simulink model "Overtaking_Integrated"  (R2020b)
settings: Solver=ode23tb  StartTime=0.0  StopTime=25  FixedStep=.01  RelTol=5e-3  EnableMultiTasking=on
InitFcn:
  | %SimulationParameters;
StartFcn:
  | %tic
StopFcn:
  | %toc
  | save(['SimOutputs\' char(datetime('now','Format','y_M_d_HH_mm_ss')) '_' 'sim_out.mat'], 'logsout');
model workspace (MAT data in the model file):
  DLCXref = [-3.2158 4.0142 4.2842 14.7842 29.7842 30.2842 41.7842 46.7842 56.7842]
  DLCYref = [-3.1012 -3.1012 -7.6012 -7.1012 -6.8512 -1.6012 -1.8512 -3.1012 -3.1012]
  Downshift_Speeds = [9.5625 12.9375 16.3125 19.6875 23.0625 26.4375 29.8125 33.1875 36.5625 39.9375 43.3125 46.6875 ... (28 elements, 4x7)]
  EngRevLim = 7000
  Pedal_Positions = [0.1 0.4 0.5 0.9]
  Upshift_Speeds = [12.9375 16.3125 19.6875 33 26.4375 29.8125 33.1875 52.5 39.9375 43.3125 46.6875 77.25 ... (28 elements, 4x7)]
  VEH : object (value not decoded)
values from neighbouring files (symbols this model uses):
  abortTrigger = 0.0    [AOTDataDictionary.sldd]
  Dmax = 3.0    [AOTDataDictionary.sldd]
  dt = 0.05    [AOTDataDictionary.sldd]
  egoVehLength = 4.948    [AOTDataDictionary.sldd]
  egoVehWidth = 2.009    [AOTDataDictionary.sldd]
  gamma = 0.5    [AOTDataDictionary.sldd]
  inflationFactor = 1.1    [AOTDataDictionary.sldd]
  inflexPoint = 0.0    [AOTDataDictionary.sldd]
  L = 3.705    [AOTDataDictionary.sldd]
  npcVehLength = 4.848    [AOTDataDictionary.sldd]
  npcVehWidth = 1.842    [AOTDataDictionary.sldd]
  plotSampleTime = 0.1    [AOTDataDictionary.sldd]
  SenseResolution = 0.1    [AOTDataDictionary.sldd]
  XSenseRange = 20.0    [AOTDataDictionary.sldd]
  YSenseRange = 20.0    [AOTDataDictionary.sldd]
symbols that are objects in the model workspace (value not decoded): VEH
undefined symbols (not defined in the file or in its folder): driving
libraries: simulink x10, drivingscenarioandsensors x5, autolibutils x4, sim3dautolib x3, sim3dlib x2, autolibshared x1, vehdynlibdriver x1, vehdynlibscenariocommon x1, pid_lib x1, vehdynlibsens x1
(part 2 of 3)

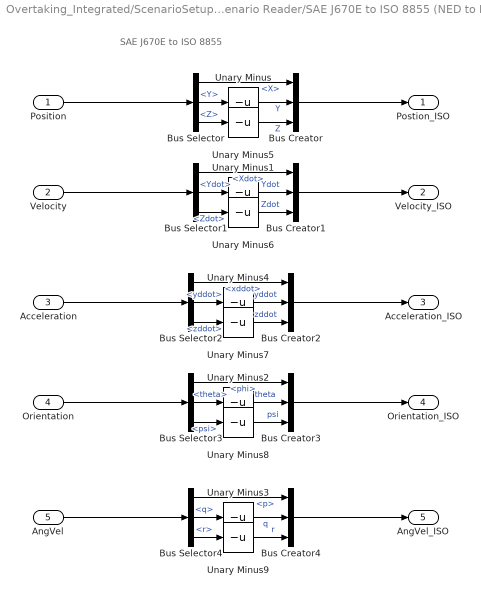
== system Overtaking_Integrated/ScenarioSetup/Scenario Reader/SAE J670E to ISO 8855 (NED to NWU)1 ==
  note: SAE J670E to ISO 8855
  Position : Inport  Unit=m
  Velocity : Inport  Port=2  Unit=m/s
  Acceleration : Inport  Port=3  Unit=m/s^2
  Orientation : Inport  Port=4  Unit=rad
  AngVel : Inport  Port=5  Unit=rad/s
  Bus Creator{,1..4} (5 alike) : BusCreator  Inputs=3
  Bus Selector : BusSelector  OutputSignals=X,Y,Z
  Bus Selector1 : BusSelector  OutputSignals=Xdot,Ydot,Zdot
  Bus Selector2 : BusSelector  OutputSignals=xddot,yddot,zddot
  Bus Selector3 : BusSelector  OutputSignals=phi,theta,psi
  Bus Selector4 : BusSelector  OutputSignals=p,q,r
  Unary Minus{,1..9} (10 alike) : UnaryMinus
  Postion_ISO : Outport  Unit=m  VectorParamsAs1DForOutWhenUnconnected=off
  Velocity_ISO : Outport  Port=2  Unit=m/s  VectorParamsAs1DForOutWhenUnconnected=off  LockScale=on
  Acceleration_ISO : Outport  Port=3  Unit=m/s^2  VectorParamsAs1DForOutWhenUnconnected=off
  Orientation_ISO : Outport  Port=4  Unit=rad  VectorParamsAs1DForOutWhenUnconnected=off
  AngVel_ISO : Outport  Port=5  Unit=rad/s  VectorParamsAs1DForOutWhenUnconnected=off
  wires:
  Bus Creator2/1 -> Acceleration_ISO/1
  Position/1 -> Bus Selector/1
  Bus Selector/2 -> Unary Minus/1  "<Y>"
  Bus Selector/1 -> Bus Creator/1  "<X>"
  Unary Minus/1 -> Bus Creator/2  "Y"
  Bus Selector/3 -> Unary Minus5/1  "<Z>"
  Unary Minus5/1 -> Bus Creator/3  "Z"
  Bus Creator/1 -> Postion_ISO/1
  Unary Minus6/1 -> Bus Creator1/3  "Zdot"
  Unary Minus1/1 -> Bus Creator1/2  "Ydot"
  Bus Selector1/2 -> Unary Minus1/1  "<Ydot>"
  Bus Selector1/1 -> Bus Creator1/1  "<Xdot>"
  Bus Selector1/3 -> Unary Minus6/1  "<Zdot>"
  Velocity/1 -> Bus Selector1/1
  Bus Creator1/1 -> Velocity_ISO/1
  Unary Minus7/1 -> Bus Creator2/3  "zddot"
  Unary Minus4/1 -> Bus Creator2/2  "yddot"
  Bus Selector2/2 -> Unary Minus4/1  "<yddot>"
  Bus Selector2/1 -> Bus Creator2/1  "<xddot>"
  Bus Selector2/3 -> Unary Minus7/1  "<zddot>"
  Acceleration/1 -> Bus Selector2/1
  Bus Selector3/3 -> Unary Minus8/1  "<psi>"
  Bus Selector3/2 -> Unary Minus2/1  "<theta>"
  Unary Minus2/1 -> Bus Creator3/2  "theta"
  Bus Selector3/1 -> Bus Creator3/1  "<phi>"
  Unary Minus8/1 -> Bus Creator3/3  "psi"
  Orientation/1 -> Bus Selector3/1
  Bus Creator3/1 -> Orientation_ISO/1
  Bus Selector4/1 -> Bus Creator4/1  "<p>"
  Bus Creator4/1 -> AngVel_ISO/1
  Bus Selector4/2 -> Unary Minus3/1  "<q>"
  Unary Minus9/1 -> Bus Creator4/3  "r"
  Unary Minus3/1 -> Bus Creator4/2  "q"
  Bus Selector4/3 -> Unary Minus9/1  "<r>"
  AngVel/1 -> Bus Selector4/1

== system Overtaking_Integrated/Subsystem3/Driver Commands/Driver Commands ==
  VehRef : Inport
  VehFdbk : Inport  Port=2
  SteerCmd : Inport  Port=3
  Accel : Inport  Port=4
  Brake : Inport  Port=5
  Gear : Inport  Port=6
  Longitudinal Driver : Subsystem  VariantControl=0
  Open Loop Constant Radius : Subsystem  VariantControl=2
  Predictive Driver : Subsystem  VariantControl=1
  " Driver" : Outport  VectorParamsAs1DForOutWhenUnconnected=off

== system Overtaking_Integrated/Vehicle Plant/Controllers/Active Differential Control ==
  note: 1) Add Subsystem or Model blocks as valid variant choices.
      | 2) You cannot connect blocks at this level. At simulation, connectivity is automatically
      | determined, based on the active variant and port name matching.
  Accel : Inport
  BrkCmd : Inport  Port=2
  Steer : Inport  Port=3
  GearFdbk : Inport  Port=4
  Omega : Inport  Port=5  Unit=rad/s
  axayaz : Inport  Port=6
  pqr : Inport  Port=7
  No Control : Subsystem  VariantControl=0
  Rear Diff Controller : Subsystem  TreatAsAtomicUnit=on  SystemSampleTime=.01  VariantControl=1
  DiffPrsCmd : Outport  VectorParamsAs1DForOutWhenUnconnected=off
  TrqCmd : Outport  Port=2  VectorParamsAs1DForOutWhenUnconnected=off

== system Overtaking_Integrated/Vehicle Plant/Controllers/Brake Controller ==
  BrkCmd : Inport
  Omega : Inport  Port=2
  kappa : Inport  Port=3
  Abs : Abs  ZeroCross=off
  Brake Pressure Control : Subsystem  Variant=on  VariantControlMode=label  LabelModeActiveChoice=0
  Constant1 : Constant  Value=-20
  Gain3 : Gain
  Integrator2 : Integrator  LimitOutput=on  UpperSaturationLimit=1  LowerSaturationLimit=0
  Saturation : Saturate  UpperLimit=1  LowerLimit=0  ZeroCross=off
  Switch1 : Switch  Criteria=u2 > Threshold  Threshold=.1
  Vector Concatenate2 : Concatenate  NumInputs=4
  BrkPrsCmd : Outport  VectorParamsAs1DForOutWhenUnconnected=off
  wires:
  Constant1/1 -> Switch1/3
  Gain3/1 -> Switch1/1
  Saturation/1 -> Brake Pressure Control/3(<Kappa>)  "Kappa"
  Brake Pressure Control/1(BrkPrsCmd) -> BrkPrsCmd/1
  kappa/1 -> Abs/1
  Integrator2/1 -> Vector Concatenate2/4, Vector Concatenate2/3, Vector Concatenate2/2, Vector Concatenate2/1
  Omega/1 -> Brake Pressure Control/2(Omega)
  Abs/1 -> Saturation/1
  Vector Concatenate2/1 -> Brake Pressure Control/1(Pref)  "Reference P"
  BrkCmd/1 -> Switch1/2, Gain3/1
  Switch1/1 -> Integrator2/1

== system Overtaking_Integrated/Vehicle Plant/Controllers/ECU ==
  DiffTrqCmd : Inport
  <Accel> : Inport  Port=2
  EngSpd : Inport  Port=3
  First Order Hold : FirstOrderHold  ErrorTolerance=100
  Torque Cmd : Subsystem  TreatAsAtomicUnit=on  SystemSampleTime=.01
  EngTrqCmd : Outport  VectorParamsAs1DForOutWhenUnconnected=off
  wires:
  First Order Hold/1 -> EngTrqCmd/1
  DiffTrqCmd/1 -> Torque Cmd/1(DiffTrqCmd)
  <Accel>/1 -> Torque Cmd/2(<Accel>)
  EngSpd/1 -> Torque Cmd/3(EngSpd)
  Torque Cmd/1(EngTrqCmd) -> First Order Hold/1

== system Overtaking_Integrated/Vehicle Plant/Controllers/Transmission Controller ==
  Accel : Inport
  BrkCmd : Inport  Port=2
  GearReq : Inport  Port=3
  EngSpd : Inport  Port=4
  Omega : Inport  Port=5  Unit=rad/s
  UpReq : Inport  Port=6
  DownReq : Inport  Port=7  Unit=rad/s
  Driver - No Clutch : Subsystem  VariantControl=1
  PRNDL Controller : Subsystem  VariantControl=3
  Paddles : Subsystem  VariantControl=2
  Transmission Controller : Subsystem  VariantControl=0
  " Gear" : Outport  VectorParamsAs1DForOutWhenUnconnected=off

== system Overtaking_Integrated/Vehicle Plant/Environment/Ground Feedback ==
  Friction : Inport
  3D Engine : Subsystem  VariantControl=1
  Constant : Subsystem  VariantControl=0
  Ground : Outport  VectorParamsAs1DForOutWhenUnconnected=off

== system Overtaking_Integrated/Vehicle Plant/Passenger Vehicle/Body, Suspension, Wheels ==
  note: 1) Add Subsystem or Model blocks as valid variant choices.
      | 2) You cannot connect blocks at this level. At simulation, connectivity is automatically
      | determined, based on the active variant and port name matching.
  WindXYZ : Inport
  Ground : Inport  Port=2  PortDimensions=4
  Friction : Inport  Port=3  PortDimensions=4
  WhlAng : Inport  Port=4
  AxlTrq : Inport  Port=5
  BrkPrs : Inport  Port=6
  PassVeh14DOF : ModelReference  DisableCoverage=on  ModelNameDialog=PassVeh14DOF  VariantControl=3  ModelReferenceVersion=2.28
  PassVeh7DOF : ModelReference  ModelNameDialog=PassVeh7DOF  SimulationMode=Normal  VariantControl=1  ModelReferenceVersion=2.94
  Veh : Outport  VectorParamsAs1DForOutWhenUnconnected=off
  Wheels : Outport  Port=2  VectorParamsAs1DForOutWhenUnconnected=off

== system Overtaking_Integrated/Vehicle Plant/Passenger Vehicle/Chassis Input ==
  Env : Inport
  Driveline : Inport  Port=2
  Bus Selector1 : BusSelector  OutputSignals=Gnd.z.G_FL_z,Gnd.z.G_FR_z,Gnd.z.G_RL_z,Gnd.z.G_RR_z
  Bus Selector2 : BusSelector  OutputSignals=Wind
  Bus Selector3 : BusSelector  OutputSignals=Gnd.mu.mu_FL,Gnd.mu.mu_FR,Gnd.mu.mu_RL,Gnd.mu.mu_RR
  Bus Selector4 : BusSelector  OutputSignals=WhlAng,AxlTrq,BrkPrs
  Vector Concatenate : Concatenate  NumInputs=4
  Vector Concatenate1 : Concatenate  NumInputs=4
  Wind : Outport  VectorParamsAs1DForOutWhenUnconnected=off
  Gnd : Outport  Port=2  VectorParamsAs1DForOutWhenUnconnected=off
  mu : Outport  Port=3  VectorParamsAs1DForOutWhenUnconnected=off
  WhlAng : Outport  Port=4  VectorParamsAs1DForOutWhenUnconnected=off
  AxlTrq : Outport  Port=5  VectorParamsAs1DForOutWhenUnconnected=off
  BrkPrs : Outport  Port=6  VectorParamsAs1DForOutWhenUnconnected=off
  wires:
  Env/1 -> Bus Selector3/1, Bus Selector1/1, Bus Selector2/1
  Bus Selector2/1 -> Wind/1  "<Wind>"
  Bus Selector3/1 -> Vector Concatenate/1  "<mu_FL>"
  Bus Selector3/2 -> Vector Concatenate/2  "<mu_FR>"
  Bus Selector3/3 -> Vector Concatenate/3  "<mu_RL>"
  Bus Selector3/4 -> Vector Concatenate/4  "<mu_RR>"
  Vector Concatenate/1 -> mu/1
  Bus Selector1/1 -> Vector Concatenate1/1  "<G_FL_z>"
  Bus Selector1/2 -> Vector Concatenate1/2  "<G_FR_z>"
  Bus Selector1/3 -> Vector Concatenate1/3  "<G_RL_z>"
  Bus Selector1/4 -> Vector Concatenate1/4  "<G_RR_z>"
  Vector Concatenate1/1 -> Gnd/1
  Driveline/1 -> Bus Selector4/1
  Bus Selector4/2 -> AxlTrq/1  "<AxlTrq>"
  Bus Selector4/1 -> WhlAng/1  "<WhlAng>"
  Bus Selector4/3 -> BrkPrs/1  "<BrkPrs>"

== system Overtaking_Integrated/Vehicle Plant/Passenger Vehicle/Chassis Output ==
  Veh : Inport
  Wheels : Inport  Port=2
  Out Bus Element4 : Outport  PortName=VehFdbk
  Out Bus Element1 : Outport  Port=2  PortName=WheelsFdbk
  wires:
  Veh/1 -> Out Bus Element4/1
  Wheels/1 -> Out Bus Element1/1

== system Overtaking_Integrated/Vehicle Plant/Passenger Vehicle/Driveline Input ==
  Cntrl : Inport
  Driver : Inport  Port=2
  EngTrqCmd : Inport  Port=3
  Wheels : Inport  Port=4
  Bus Selector1 : BusSelector  OutputSignals=SteerCmd
  Bus Selector2 : BusSelector  OutputSignals=TireFrame.Omega
  Bus Selector3 : BusSelector  OutputSignals=Transmission.GearCmd,Brake.BrkPrsCmd,Diff.DiffPrsCmd
  Bus Selector4 : BusSelector  OutputSignals=EngTrq
  Data Type Conversion : DataTypeConversion
  Steer : Outport  VectorParamsAs1DForOutWhenUnconnected=off
  EngTrq : Outport  Port=2  VectorParamsAs1DForOutWhenUnconnected=off
  GearCmd : Outport  Port=3  VectorParamsAs1DForOutWhenUnconnected=off
  BrkPrsCmd : Outport  Port=4  VectorParamsAs1DForOutWhenUnconnected=off
  Omega : Outport  Port=5  VectorParamsAs1DForOutWhenUnconnected=off
  DiffPrsCmd : Outport  Port=6  VectorParamsAs1DForOutWhenUnconnected=off
  wires:
  Cntrl/1 -> Bus Selector3/1
  Bus Selector3/1 -> Data Type Conversion/1  "<GearCmd>"
  Driver/1 -> Bus Selector1/1
  Wheels/1 -> Bus Selector2/1
  Bus Selector2/1 -> Omega/1  "<Omega>"
  Bus Selector3/2 -> BrkPrsCmd/1  "<BrkPrsCmd>"
  EngTrqCmd/1 -> Bus Selector4/1
  Bus Selector1/1 -> Steer/1  "<SteerCmd>"
  Bus Selector4/1 -> EngTrq/1  "<EngTrq>"
  Bus Selector3/3 -> DiffPrsCmd/1  "<DiffPrsCmd>"
  Data Type Conversion/1 -> GearCmd/1

== system Overtaking_Integrated/Vehicle Plant/Passenger Vehicle/Driveline Output ==
  WhlAng : Inport
  AxlTrq : Inport  Port=2
  BrkPrs : Inport  Port=3
  EngSpd : Inport  Port=4
  PropShftSpd : Inport  Port=5
  StrWhlTrq : Inport  Port=6
  Gear : Inport  Port=7
  Bus Creator1 : BusCreator  Inputs=6
  Bus Creator2 : BusCreator  Inputs=1
  Driveline : Outport  VectorParamsAs1DForOutWhenUnconnected=off
  Steering : Outport  Port=2  VectorParamsAs1DForOutWhenUnconnected=off
  wires:
  Bus Creator1/1 -> Driveline/1  "Driveline"
  PropShftSpd/1 -> Bus Creator1/5  "PropShftSpd"
  AxlTrq/1 -> Bus Creator1/2  "AxlTrq"
  WhlAng/1 -> Bus Creator1/1  "WhlAng"
  EngSpd/1 -> Bus Creator1/4  "EngSpd"
  BrkPrs/1 -> Bus Creator1/3  "BrkPrs"
  StrWhlTrq/1 -> Bus Creator2/1  "StrWhlTrq"
  Bus Creator2/1 -> Steering/1  "Steering"
  Gear/1 -> Bus Creator1/6  "Gear"

== system Overtaking_Integrated/Vehicle Plant/Passenger Vehicle/Engine ==
  note: 1) Add Subsystem or Model blocks as valid variant choices.
      | 2) You cannot connect blocks at this level. At simulation, connectivity is automatically
      | determined, based on the active variant and port name matching.
  TrqCmd : Inport
  EngSpd : Inport  Port=2  Unit=rad/s
  Ideal Mapped Engine : ModelReference  DisableCoverage=on  ModelNameDialog=SiMappedEngineV  VariantControl=0  ModelReferenceVersion=1.335
  EngTrq : Outport  VectorParamsAs1DForOutWhenUnconnected=off

== system Overtaking_Integrated/Vehicle Plant/Passenger Vehicle/Engine Input ==
  Cntrl : Inport
  Driveline : Inport  Port=2
  Bus Selector : BusSelector  OutputSignals=ECU.EngTrqCmd
  Bus Selector1 : BusSelector  OutputSignals=EngSpd
  EngTrqCmd : Outport  VectorParamsAs1DForOutWhenUnconnected=off
  EngSpd : Outport  Port=2  VectorParamsAs1DForOutWhenUnconnected=off
  wires:
  Driveline/1 -> Bus Selector1/1
  Cntrl/1 -> Bus Selector/1
  Bus Selector/1 -> EngTrqCmd/1  "<EngTrqCmd>"
  Bus Selector1/1 -> EngSpd/1  "<EngSpd>"

== system Overtaking_Integrated/Vehicle Plant/Passenger Vehicle/Engine Output ==
  "EngTrq " : Inport
  Bus Creator : BusCreator  Inputs=1
  Eng : Outport  VectorParamsAs1DForOutWhenUnconnected=off
  wires:
  "EngTrq "/1 -> Bus Creator/1  "EngTrq"
  Bus Creator/1 -> Eng/1

== system Overtaking_Integrated/Vehicle Plant/Passenger Vehicle/Pedal Cluster Input ==
  Driver : Inport
  Driveline : Inport  Port=2
  Steering : Inport  Port=3
  Bus Selector : BusSelector  OutputSignals=SteerCmd,AccelCmd,DecelCmd,GearCmd
  Bus Selector1 : BusSelector  OutputSignals=BrkPrs
  Bus Selector2 : BusSelector  OutputSignals=StrWhlTrq
  SteerCmd : Outport  VectorParamsAs1DForOutWhenUnconnected=off
  AccelCmd : Outport  Port=2  VectorParamsAs1DForOutWhenUnconnected=off
  DecelCmd : Outport  Port=3  VectorParamsAs1DForOutWhenUnconnected=off
  GearCmd : Outport  Port=4  VectorParamsAs1DForOutWhenUnconnected=off
  BrkPrs : Outport  Port=5  VectorParamsAs1DForOutWhenUnconnected=off
  StrWhlTrq : Outport  Port=6  VectorParamsAs1DForOutWhenUnconnected=off
  wires:
  Bus Selector/2 -> AccelCmd/1  "<AccelCmd>"
  Driver/1 -> Bus Selector/1
  Bus Selector/3 -> DecelCmd/1  "<DecelCmd>"
  Bus Selector/4 -> GearCmd/1  "<GearCmd>"
  Bus Selector/1 -> SteerCmd/1  "<SteerCmd>"
  Driveline/1 -> Bus Selector1/1
  Bus Selector1/1 -> BrkPrs/1  "<BrkPrs>"
  Steering/1 -> Bus Selector2/1
  Bus Selector2/1 -> StrWhlTrq/1  "<StrWhlTrq>"

== system Overtaking_Integrated/Vehicle Plant/Passenger Vehicle/Pedal Cluster Output ==
  SteerFdbk : Inport
  AccFdbk : Inport  Port=2
  DecelFdbk : Inport  Port=3
  GearFdbk : Inport  Port=4
  Bus Creator1 : BusCreator  Inputs=4
  Signal Specification : SignalSpecification  Unit=rad
  Signal Specification1 : SignalSpecification  Unit=1
  Signal Specification2 : SignalSpecification  Unit=1
  Signal Specification3 : SignalSpecification  Unit=1
  OperatorFdbk : Outport
  wires:
  Signal Specification1/1 -> Bus Creator1/2  "AccFdbk"
  Signal Specification3/1 -> Bus Creator1/4  "GearFdbk"
  AccFdbk/1 -> Signal Specification1/1
  DecelFdbk/1 -> Signal Specification2/1
  GearFdbk/1 -> Signal Specification3/1
  Signal Specification/1 -> Bus Creator1/1  "SteerFdbk"
  SteerFdbk/1 -> Signal Specification/1
  Bus Creator1/1 -> OperatorFdbk/1
  Signal Specification2/1 -> Bus Creator1/3  "DecelFdbk"

== system Overtaking_Integrated/Vehicle Plant/Passenger Vehicle/Pedal Cluster and Cabin ==
  note: Placeholder for introducing faults, detailed actuator behavior,
      | interactions of other systems with a human interface such
      | as changes in power steering and braking assistance.
  SteerCmd : Inport
  AccCmd : Inport  Port=2
  DecelCmd : Inport  Port=3
  GearCmd : Inport  Port=4
  BrkPrs : Inport  Port=5
  StrWhlTrq : Inport  Port=6
  Terminator : Terminator
  Terminator1 : Terminator
  SteerFdbk : Outport
  AccFdbk : Outport  Port=2
  DecelFdbk : Outport  Port=3
  GearFdbk : Outport  Port=4
  wires:
  SteerCmd/1 -> SteerFdbk/1
  AccCmd/1 -> AccFdbk/1
  DecelCmd/1 -> DecelFdbk/1
  GearCmd/1 -> GearFdbk/1
  BrkPrs/1 -> Terminator/1
  StrWhlTrq/1 -> Terminator1/1

== system Overtaking_Integrated/Vehicle Plant/Passenger Vehicle/Steering, Transmission, Driveline and Brakes ==
  note: 1) Add Subsystem or Model blocks as valid variant choices.
      | 2) You cannot connect blocks at this level. At simulation, connectivity is automatically
      | determined, based on the active variant and port name matching.
  SteerHWCmd : Inport
  EngTrq : Inport  Port=2
  GearCmd : Inport  Port=3  OutDataTypeStr=int8
  BrkPrsCmd : Inport  Port=4  PortDimensions=4
  Omega : Inport  Port=5
  DiffPrsCmd : Inport  Port=6
  Driveline Ideal Fixed Gear : ModelReference  DisableCoverage=on  ModelNameDialog=Driveline  VariantControl=0  ModelReferenceVersion=1.238
  WhlAng : Outport  VectorParamsAs1DForOutWhenUnconnected=off
  AxlTrq : Outport  Port=2  VectorParamsAs1DForOutWhenUnconnected=off
  BrkPrs : Outport  Port=3  PortDimensions=4  VectorParamsAs1DForOutWhenUnconnected=off
  EngSpd : Outport  Port=4  Unit=rad/s  VectorParamsAs1DForOutWhenUnconnected=off
  PropShftSpd : Outport  Port=5  VectorParamsAs1DForOutWhenUnconnected=off
  StrWhlTrq : Outport  Port=6  VectorParamsAs1DForOutWhenUnconnected=off
  Gear : Outport  Port=7  VectorParamsAs1DForOutWhenUnconnected=off

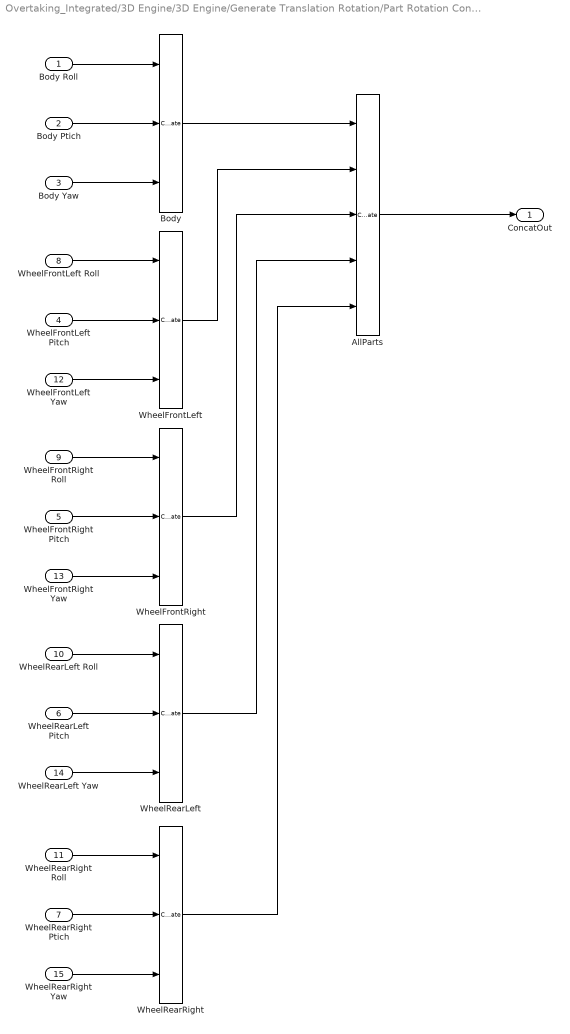
== system Overtaking_Integrated/3D Engine/3D Engine/Generate Translation Rotation/Part Rotation Concatenation ==
  Body Roll : Inport
  Body Ptich : Inport  Port=2
  Body Yaw : Inport  Port=3
  WheelFrontLeft Pitch : Inport  Port=4
  WheelFrontRight Pitch : Inport  Port=5
  WheelRearLeft Pitch : Inport  Port=6
  WheelRearRight Ptich : Inport  Port=7
  WheelFrontLeft Roll : Inport  Port=8
  WheelFrontRight Roll : Inport  Port=9
  WheelRearLeft Roll : Inport  Port=10
  WheelRearRight Roll : Inport  Port=11
  WheelFrontLeft Yaw : Inport  Port=12
  WheelFrontRight Yaw : Inport  Port=13
  WheelRearLeft Yaw : Inport  Port=14
  WheelRearRight Yaw : Inport  Port=15
  AllParts : Concatenate  NumInputs=5  Mode=Multidimensional array
  Body : Concatenate  NumInputs=3  Mode=Multidimensional array  ConcatenateDimension=2
  WheelFrontLeft : Concatenate  NumInputs=3  Mode=Multidimensional array  ConcatenateDimension=2
  WheelFrontRight : Concatenate  NumInputs=3  Mode=Multidimensional array  ConcatenateDimension=2
  WheelRearLeft : Concatenate  NumInputs=3  Mode=Multidimensional array  ConcatenateDimension=2
  WheelRearRight : Concatenate  NumInputs=3  Mode=Multidimensional array  ConcatenateDimension=2
  ConcatOut : Outport  VectorParamsAs1DForOutWhenUnconnected=off
  wires:
  Body Yaw/1 -> Body/3
  WheelFrontLeft Yaw/1 -> WheelFrontLeft/3
  WheelFrontLeft/1 -> AllParts/2
  Body/1 -> AllParts/1
  WheelRearLeft/1 -> AllParts/4
  WheelFrontRight/1 -> AllParts/3
  WheelRearRight Yaw/1 -> WheelRearRight/3
  WheelRearLeft Yaw/1 -> WheelRearLeft/3
  AllParts/1 -> ConcatOut/1
  WheelRearRight/1 -> AllParts/5
  WheelFrontRight Yaw/1 -> WheelFrontRight/3
  Body Roll/1 -> Body/1
  Body Ptich/1 -> Body/2
  WheelFrontLeft Pitch/1 -> WheelFrontLeft/2
  WheelFrontLeft Roll/1 -> WheelFrontLeft/1
  WheelFrontRight Roll/1 -> WheelFrontRight/1
  WheelFrontRight Pitch/1 -> WheelFrontRight/2
  WheelRearLeft Roll/1 -> WheelRearLeft/1
  WheelRearLeft Pitch/1 -> WheelRearLeft/2
  WheelRearRight Roll/1 -> WheelRearRight/1
  WheelRearRight Ptich/1 -> WheelRearRight/2

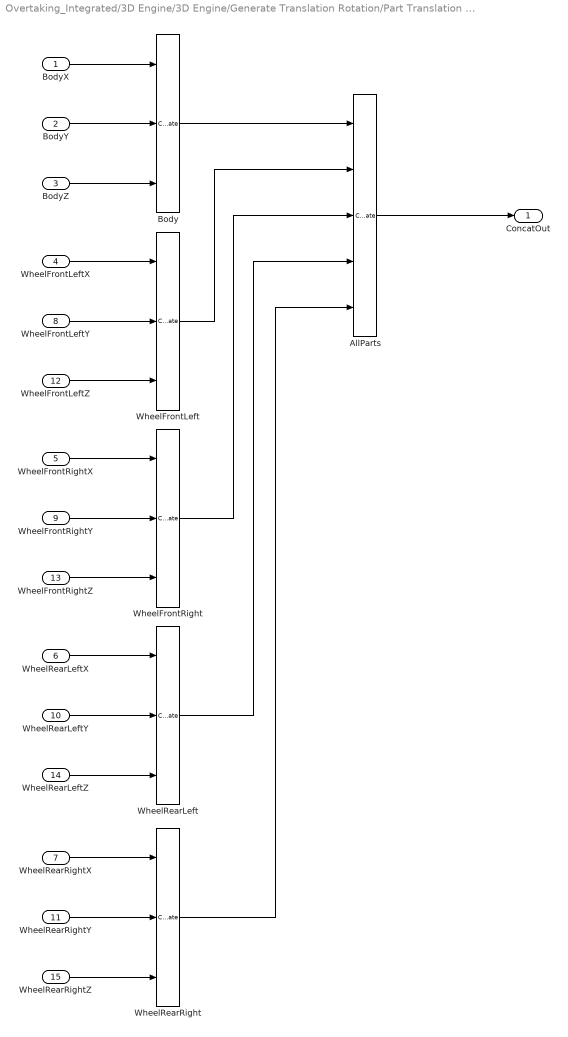
== system Overtaking_Integrated/3D Engine/3D Engine/Generate Translation Rotation/Part Translation Concatenation ==
  BodyX : Inport
  BodyY : Inport  Port=2
  BodyZ : Inport  Port=3
  WheelFrontLeftX : Inport  Port=4
  WheelFrontRightX : Inport  Port=5
  WheelRearLeftX : Inport  Port=6
  WheelRearRightX : Inport  Port=7
  WheelFrontLeftY : Inport  Port=8
  WheelFrontRightY : Inport  Port=9
  WheelRearLeftY : Inport  Port=10
  WheelRearRightY : Inport  Port=11
  WheelFrontLeftZ : Inport  Port=12
  WheelFrontRightZ : Inport  Port=13
  WheelRearLeftZ : Inport  Port=14
  WheelRearRightZ : Inport  Port=15
  AllParts : Concatenate  NumInputs=5  Mode=Multidimensional array
  Body : Concatenate  NumInputs=3  Mode=Multidimensional array  ConcatenateDimension=2
  WheelFrontLeft : Concatenate  NumInputs=3  Mode=Multidimensional array  ConcatenateDimension=2
  WheelFrontRight : Concatenate  NumInputs=3  Mode=Multidimensional array  ConcatenateDimension=2
  WheelRearLeft : Concatenate  NumInputs=3  Mode=Multidimensional array  ConcatenateDimension=2
  WheelRearRight : Concatenate  NumInputs=3  Mode=Multidimensional array  ConcatenateDimension=2
  ConcatOut : Outport  VectorParamsAs1DForOutWhenUnconnected=off
  wires:
  BodyX/1 -> Body/1
  BodyZ/1 -> Body/3
  WheelFrontLeftX/1 -> WheelFrontLeft/1
  WheelFrontLeftZ/1 -> WheelFrontLeft/3
  WheelFrontLeftY/1 -> WheelFrontLeft/2
  BodyY/1 -> Body/2
  WheelFrontLeft/1 -> AllParts/2
  WheelRearRightX/1 -> WheelRearRight/1
  Body/1 -> AllParts/1
  WheelRearLeft/1 -> AllParts/4
  WheelFrontRight/1 -> AllParts/3
  WheelRearRightZ/1 -> WheelRearRight/3
  WheelFrontRightY/1 -> WheelFrontRight/2
  WheelFrontRightX/1 -> WheelFrontRight/1
  WheelRearRightY/1 -> WheelRearRight/2
  WheelRearLeftZ/1 -> WheelRearLeft/3
  AllParts/1 -> ConcatOut/1
  WheelRearLeftY/1 -> WheelRearLeft/2
  WheelRearRight/1 -> AllParts/5
  WheelRearLeftX/1 -> WheelRearLeft/1
  WheelFrontRightZ/1 -> WheelFrontRight/3

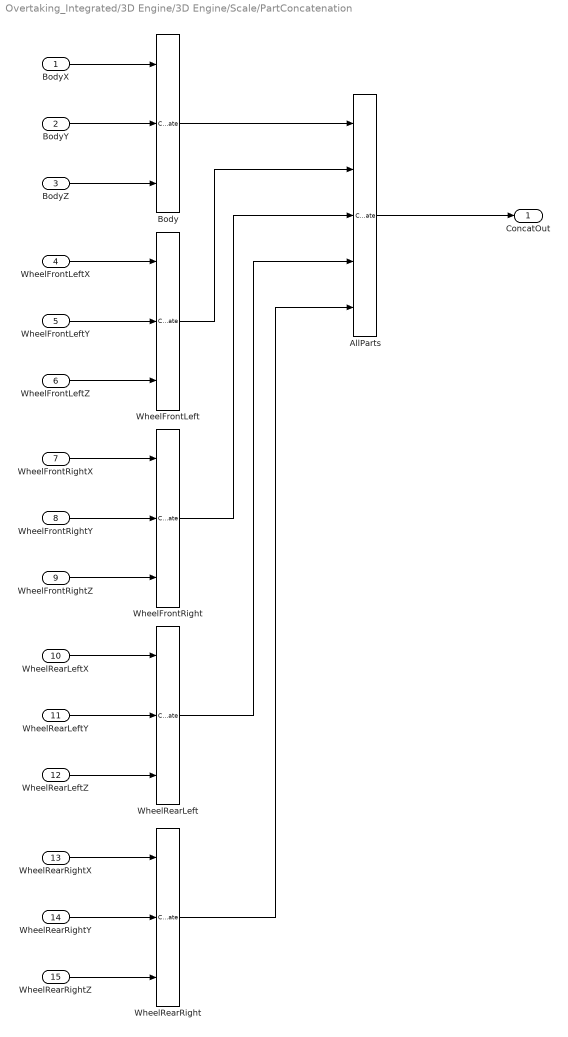
== system Overtaking_Integrated/3D Engine/3D Engine/Scale/PartConcatenation ==
  BodyX : Inport
  BodyY : Inport  Port=2
  BodyZ : Inport  Port=3
  WheelFrontLeftX : Inport  Port=4
  WheelFrontLeftY : Inport  Port=5
  WheelFrontLeftZ : Inport  Port=6
  WheelFrontRightX : Inport  Port=7
  WheelFrontRightY : Inport  Port=8
  WheelFrontRightZ : Inport  Port=9
  WheelRearLeftX : Inport  Port=10
  WheelRearLeftY : Inport  Port=11
  WheelRearLeftZ : Inport  Port=12
  WheelRearRightX : Inport  Port=13
  WheelRearRightY : Inport  Port=14
  WheelRearRightZ : Inport  Port=15
  AllParts : Concatenate  NumInputs=5  Mode=Multidimensional array
  Body : Concatenate  NumInputs=3  Mode=Multidimensional array  ConcatenateDimension=2
  WheelFrontLeft : Concatenate  NumInputs=3  Mode=Multidimensional array  ConcatenateDimension=2
  WheelFrontRight : Concatenate  NumInputs=3  Mode=Multidimensional array  ConcatenateDimension=2
  WheelRearLeft : Concatenate  NumInputs=3  Mode=Multidimensional array  ConcatenateDimension=2
  WheelRearRight : Concatenate  NumInputs=3  Mode=Multidimensional array  ConcatenateDimension=2
  ConcatOut : Outport  VectorParamsAs1DForOutWhenUnconnected=off
  wires:
  BodyX/1 -> Body/1
  BodyZ/1 -> Body/3
  WheelFrontLeftX/1 -> WheelFrontLeft/1
  WheelFrontLeftZ/1 -> WheelFrontLeft/3
  WheelFrontLeftY/1 -> WheelFrontLeft/2
  BodyY/1 -> Body/2
  WheelFrontLeft/1 -> AllParts/2
  WheelRearRightX/1 -> WheelRearRight/1
  Body/1 -> AllParts/1
  WheelRearLeft/1 -> AllParts/4
  WheelFrontRight/1 -> AllParts/3
  WheelRearRightZ/1 -> WheelRearRight/3
  WheelFrontRightY/1 -> WheelFrontRight/2
  WheelFrontRightX/1 -> WheelFrontRight/1
  WheelRearRightY/1 -> WheelRearRight/2
  WheelRearLeftZ/1 -> WheelRearLeft/3
  AllParts/1 -> ConcatOut/1
  WheelRearLeftY/1 -> WheelRearLeft/2
  WheelRearRight/1 -> AllParts/5
  WheelRearLeftX/1 -> WheelRearLeft/1
  WheelFrontRightZ/1 -> WheelFrontRight/3

== system Overtaking_Integrated/Subsystem3/Driver Commands/Driver Commands/Longitudinal Driver ==
  VehRef : Inport
  VehFdbk : Inport  Port=2
  Bus Creator2 : BusCreator  Inputs=5
  Bus Selector2 : BusSelector  OutputSignals=Body.BdyFrm.Cg.Vel.xdot,Body.InertFrm.Cg.Disp.X
  Bus Selector3 : BusSelector  OutputSignals=SteerOvrCmd,LngRef,LtrlRef
  Dead Zone1 : DeadZone  LowerValue=-.1  UpperValue=.1  SaturateOnIntegerOverflow=on
  Ground1 : Ground
  Ground2 : Ground
  Longitudinal Driver : autolibshared/Longitudinal Driver  extAccelOvr=off  extDecelOvr=off  extAccelHld=off  extDecelHld=off  extAccelZero=off  extDecelZero=off  cntrlType=Predictive  shftType=Reverse, Neutral, Drive  velUnits=m/s  gearOut=on  Kp=5  Ki=5  Kff=.1  Kg=0  VehVelVec=[0 100]  KffVec=[.1 .1]  KpVec=[10 10]  KiVec=[5 5]  KgVec=[0 0]  m=VEH.Mass  Kpt=3000  tau=.5  L=2  aR=200  bR=2.5  cR=.5  g=9.81  vnom=5  Kaw=1  tauerr=.1  tauPt=2  GearInit=0  tShift=.1  pdlVec=[0.1 0.4 0.5 0.9]  upShftTbl=[-1 12.9375 26.4375 39.9375 51.18749999999999 62.4375 72.84375 83.25;-1 16.3125 29.8125 43.3125 54.5624 65.8125 76.78125 87.75;-1 19.6875 33.1875 46.68749999999999 57.9375 69.1875 80.71875 92.25;-1 33 52.5 77.25 100.5 138.75 161.875 185]  dwnShftTbl=[1 9.5625 23.0625 36.5625 47.8125 59.0625 68.90625 78.75;1 12.9375 26.4375 39.9375 51.18749999999999 62.4375 72.84375 83.25;1 16.3125 29.8125 43.3125 54.562499 65.8125 76.78125 87.75;1 19.6875 33.1875 46.68749999999999 57.9375 69.1875 80.71875 92.25]  tClutch=.5  tRev=.5  tPark=120  aMode=2  UpGearVec="[0  1  2  3  4  5  6  7]"  DownGearVec="[1  2  3  4  5  6  7  8]"
      settings: SourceProductBaseCode=PW,MT,UV,VE,VP
  Mux : Mux  Inputs=3
  Signal Copy : SignalConversion  OverrideOpt=off
  Terminator1 : Terminator
  Driver : Outport  VectorParamsAs1DForOutWhenUnconnected=off
  wires:
  VehRef/1 -> Bus Selector3/1
  Signal Copy/1 -> Bus Creator2/1  "SteerCmd"
  Longitudinal Driver/2 -> Bus Creator2/2  "AccelCmd"
  Dead Zone1/1 -> Longitudinal Driver/2
  Bus Selector3/2 -> Longitudinal Driver/1  "<LngRef>"
  Ground1/1 -> Longitudinal Driver/3
  Bus Selector2/1 -> Dead Zone1/1  "<xdot>"
  Bus Creator2/1 -> Driver/1
  Longitudinal Driver/1 -> Terminator1/1
  Longitudinal Driver/3 -> Bus Creator2/3  "DecelCmd"
  VehFdbk/1 -> Bus Selector2/1
  Bus Selector3/1 -> Signal Copy/1  "<SteerOvrCmd>"
  Ground2/1 -> Mux/3
  Bus Selector2/2 -> Mux/1  "<X>"
  Mux/1 -> Bus Creator2/5  "Ref"
  Bus Selector3/3 -> Mux/2  "<LtrlRef>"
  Longitudinal Driver/4 -> Bus Creator2/4  "GearCmd"

== system Overtaking_Integrated/Subsystem3/Driver Commands/Driver Commands/Open Loop Constant Radius ==
  VehFdbk : Inport
  SteerCmd : Inport  Port=2
  Accel : Inport  Port=3  Unit=one
  Brake : Inport  Port=4  Unit=1
  Gear : Inport  Port=5  Unit=1
  Bus Creator1 : BusCreator  Inputs=4
  Signal Specification : SignalSpecification  Unit=rad
  Signal Specification1 : SignalSpecification  Unit=1
  Signal Specification2 : SignalSpecification  Unit=1
  Signal Specification3 : SignalSpecification  Unit=1
  Terminator : Terminator
  Unit Conversion{,1..3} (4 alike) : UnitConversion
  Driver : Outport  VectorParamsAs1DForOutWhenUnconnected=off
  wires:
  Unit Conversion3/1 -> Signal Specification3/1
  Unit Conversion2/1 -> Signal Specification2/1
  Unit Conversion/1 -> Signal Specification/1
  Bus Creator1/1 -> Driver/1
  Accel/1 -> Unit Conversion1/1
  VehFdbk/1 -> Terminator/1
  SteerCmd/1 -> Unit Conversion/1
  Unit Conversion1/1 -> Signal Specification1/1
  Brake/1 -> Unit Conversion2/1
  Gear/1 -> Unit Conversion3/1
  Signal Specification/1 -> Bus Creator1/1  "SteerCmd"
  Signal Specification1/1 -> Bus Creator1/2  "AccelCmd"
  Signal Specification2/1 -> Bus Creator1/3  "DecelCmd"
  Signal Specification3/1 -> Bus Creator1/4  "GearCmd"

== system Overtaking_Integrated/Subsystem3/Driver Commands/Driver Commands/Predictive Driver ==
  VehRef : Inport
  VehFdbk : Inport  Port=2
  Bus Creator1 : BusCreator  Inputs=5
  Bus Selector : BusSelector  OutputSignals=Body.BdyFrm.Cg.Vel.xdot,Body.InertFrm.Cg.Disp.Y,Body.BdyFrm.Cg.Vel.ydot,Body.InertFrm.Cg.Ang.psi,Body.BdyFrm.Cg.AngVel.r,Body.InertFrm.Cg.Disp.X
  Bus Selector1 : BusSelector  OutputSignals=LngRef,LtrlRef,EnblSteerCmd,SteerOvrCmd,AccelZero
  Dead Zone : DeadZone  LowerValue=-.5  UpperValue=.5  ZeroCross=off  SaturateOnIntegerOverflow=on
  Ground : Ground
  Ground1 : Ground
  Linear Predictive Driver : vehdynlibdriver/Predictive Driver  extAccelOvr=off  extDecelOvr=off  extAccelHld=off  extDecelHld=off  extAccelZero=on  extDecelZero=off  extSteerOvr=on  extSteerHld=off  extSteerZero=off  cntrlType=Predictive  cntrlTypeLat=Predictive  shftType=Reverse, Neutral, Drive  coordMode=SAE J670 (Z-down)  velUnits=m/s  angUnits=rad  gearOut=on  steerOut=on  Kp=3  Ki=1  Kff=1  Kg=0  VehVelVec=[0 100]  KffVec=[.1 .1]  KpVec=[10 10]  KiVec=[5 5]  KgVec=[0 0]  vnom=5  Kaw=1  tauerr=.075  tau=.15  L=6  Kpt=15000  aR=200  bR=2.5  cR=.5  g=9.81  vecPose=off  dynamMode=on  PositionGainF=2.5  PositionGainR=2.5  YawRateGain=.2  DelayGain=.2  a=VEH.FrontAxlePositionfromCG  b=VEH.RearAxlePositionfromCG  m=VEH.Mass  Cy_f=5000  Cy_r=7000  I=VEH.YawMomentInertia  Ksteer=18  theta=40*pi/180  GearInit=0  tShift=.1  pdlVec=[0.1 0.4 0.5 0.9]  upShftTbl=[-1 12.9375 26.4375 39.9375 51.18749999999999 62.4375 72.84375 83.25;-1 16.3125 29.8125 43.3125 54.5624 65.8125 76.78125 87.75;-1 19.6875 33.1875 46.68749999999999 57.9375 69.1875 80.71875 92.25;-1 33 52.5 77.25 100.5 138.75 161.875 185]  dwnShftTbl=[-1 12.9375 26.4375 39.9375 51.18749999999999 62.4375 72.84375 83.25;-1 16.3125 29.8125 43.3125 54.5624 65.8125 76.78125 87.75;-1 19.6875 33.1875 46.68749999999999 57.9375 69.1875 80.71875 92.25;-1 33 52.5 77.25 100.5 138.75 161.875 185]  tClutch=.5  tRev=.5  tPark=120  UpGearVec="[0  1  2  3  4  5  6  7]"  DownGearVec="[1  2  3  4  5  6  7  8]"  aMode=2
      settings: SourceProductBaseCode=VE
  Mux : Mux  Inputs=3
  Terminator : Terminator
  Driver : Outport  VectorParamsAs1DForOutWhenUnconnected=off
  wires:
  Mux/1 -> Bus Creator1/5  "Ref"
  Bus Selector/6 -> Mux/1  "<X>"
  Linear Predictive Driver/5 -> Bus Creator1/4  "GearCmd"
  Bus Selector/3 -> Linear Predictive Driver/9  "<ydot>"
  Linear Predictive Driver/1 -> Terminator/1
  Bus Selector/5 -> Linear Predictive Driver/11  "<r>"
  Bus Selector1/2 -> Mux/2, Linear Predictive Driver/2  "<LtrlRef>"
  Ground1/1 -> Mux/3
  Ground/1 -> Linear Predictive Driver/6
  Bus Selector/1 -> Dead Zone/1  "<xdot>"
  Bus Selector/4 -> Linear Predictive Driver/10  "<psi>"
  Linear Predictive Driver/4 -> Bus Creator1/3  "DecelCmd"
  Dead Zone/1 -> Linear Predictive Driver/7
  VehFdbk/1 -> Bus Selector/1
  VehRef/1 -> Bus Selector1/1  "xdotref"
  Linear Predictive Driver/2 -> Bus Creator1/1  "SteerCmd"
  Bus Creator1/1 -> Driver/1
  Linear Predictive Driver/3 -> Bus Creator1/2  "AccelCmd"
  Bus Selector/2 -> Linear Predictive Driver/8  "<Y>"
  Bus Selector1/1 -> Linear Predictive Driver/1  "<LngRef>"
  Bus Selector1/5 -> Linear Predictive Driver/5  "<AccelZero>"
  Bus Selector1/3 -> Linear Predictive Driver/3  "<EnblSteerCmd>"
  Bus Selector1/4 -> Linear Predictive Driver/4  "<SteerOvrCmd>"

== system Overtaking_Integrated/Vehicle Plant/Controllers/Active Differential Control/No Control ==
  axayaz : Inport
  Steer : Inport  Port=2
  Constant : Constant  Value=0
  Constant1 : Constant  Value=0
  Terminator : Terminator
  Terminator1 : Terminator
  Vector Concatenate2 : Concatenate  NumInputs=4
  DiffPrsCmd : Outport  VectorParamsAs1DForOutWhenUnconnected=off
  TrqCmd : Outport  Port=2  VectorParamsAs1DForOutWhenUnconnected=off
  wires:
  Constant/1 -> Vector Concatenate2/1, Vector Concatenate2/4, Vector Concatenate2/3, Vector Concatenate2/2
  Steer/1 -> Terminator1/1
  Vector Concatenate2/1 -> DiffPrsCmd/1  "DiffPrsCmd"
  axayaz/1 -> Terminator/1
  Constant1/1 -> TrqCmd/1  "TrqCmd"

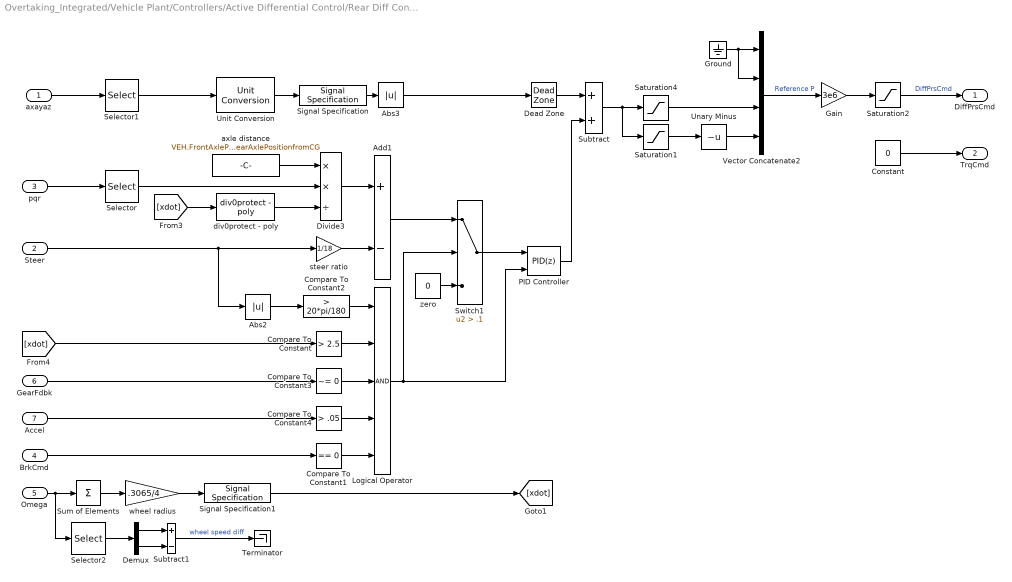
== system Overtaking_Integrated/Vehicle Plant/Controllers/Active Differential Control/Rear Diff Controller ==
  axayaz : Inport
  Steer : Inport  Port=2
  pqr : Inport  Port=3
  BrkCmd : Inport  Port=4
  Omega : Inport  Port=5  Unit=rad/s
  GearFdbk : Inport  Port=6
  Accel : Inport  Port=7
  Abs2 : Abs
  Abs3 : Abs  ZeroCross=off
  Add1 : Sum  Inputs=+-
  Compare To Constant : simulink/Logic and Bit Operations/Compare To Constant  relop=>  const=2.5  OutDataTypeStr=boolean
  Compare To Constant1 : simulink/Logic and Bit Operations/Compare To Constant  relop===  const=0  OutDataTypeStr=boolean
  Compare To Constant2 : simulink/Logic and Bit Operations/Compare To Constant  relop=>  const=20*pi/180  OutDataTypeStr=boolean
  Compare To Constant3 : simulink/Logic and Bit Operations/Compare To Constant  relop=~=  const=0  OutDataTypeStr=boolean
  Compare To Constant4 : simulink/Logic and Bit Operations/Compare To Constant  relop=>  const=.05  OutDataTypeStr=boolean
  Constant : Constant  Value=0
  Dead Zone : DeadZone  ZeroCross=off  SaturateOnIntegerOverflow=on
  Demux : Demux  Outputs=2
  Divide3 : Product  Inputs=**/
  Gain : Gain  Gain=3e6
  Ground : Ground
  Logical Operator : Logic  Inputs=5  AllPortsSameDT=off  OutDataTypeStr=boolean
  PID Controller : pid_lib/PID Controller  Controller=PID  Form=Parallel  TimeDomain=Discrete-time  UseExternalTs=off  SampleTime=-1  IntegratorMethod=Forward Euler  FilterMethod=Forward Euler  ControllerParametersSource=internal  P=1  I=.05  D=0  UseFilter=on  N=1  TunerSelectOption=Transfer Function Based (PID Tuner App)  ZeroCross=off  InitialConditionSource=internal  InitialConditionForIntegrator=0  InitialConditionForFilter=0  DifferentiatorICPrevScaledInput=0  ExternalReset=either  TrackingMode=off  Kt=1  LimitOutput=on  SatLimitsSource=internal  UpperSaturationLimit=1  LowerSaturationLimit=-1  LinearizeAsGain=on  AntiWindupMode=clamping  Kb=1  POutMin=[]  POutMax=[]  IOutMin=[]  IOutMax=[]  DOutMin=[]  DOutMax=[]  NOutMin=[]  NOutMax=[]  SumOutMin=[]  SumOutMax=[]  SaturationOutMin=[]  SaturationOutMax=[]  PParamMin=[]  PParamMax=[]  IParamMin=[]  IParamMax=[]  DParamMin=[]  DParamMax=[]  NParamMin=[]  NParamMax=[]  KbParamMin=[]  KbParamMax=[]  KtParamMin=[]  KtParamMax=[]  KbOutMin=[]  KbOutMax=[]  KtOutMin=[]  KtOutMax=[]  IntegratorOutMin=[]  IntegratorOutMax=[]  FilterOutMin=[]  FilterOutMax=[]  SumI1OutMin=[]  SumI1OutMax=[]  SumI2OutMin=[]  SumI2OutMax=[]  SumI3OutMin=[]  SumI3OutMax=[]  SumI4OutMin=[]  SumI4OutMax=[]  SumDOutMin=[]  SumDOutMax=[]  DifferentiatorOutMin=[]  DifferentiatorOutMax=[]  FilterDiffOutCoefMin=[]  FilterDiffOutCoefMax=[]  ReciprocalOutMin=[]  ReciprocalOutMax=[]  SumDenOutMin=[]  SumDenOutMax=[]  SumNumOutMin=[]  SumNumOutMax=[]  DivideOutMin=[]  DivideOutMax=[]  UdiffTsProdOutMin=[]  UdiffTsProdOutMax=[]  NTsProdOutMin=[]  NTsProdOutMax=[]  UintegralTsProdOutMin=[]  UintegralTsProdOutMax=[]  UngainTsProdOutMin=[]  UngainTsProdOutMax=[]  IntegratorContinuousStateAttributes=''  IntegratorStateMustResolveToSignalObject=off  IntegratorRTWStateStorageClass=Auto  FilterContinuousStateAttributes=''  FilterStateMustResolveToSignalObject=off  FilterRTWStateStorageClass=Auto  ParallelPVariant=InternalParameters  IdealPVariant=Disabled  IVariant=InternalParameters  DVariant=InternalParameters  IntegratorVariant=Discrete  SatVariant=Enabled  AWVariant=DiscClampingParallel  PCopyVariant=Disabled  TRVariant=Disabled  FdbkBlocksVariant=Forward  IdealPFdbkVariant=Disabled  SatFdbkVariant=Disabled  DerivativeFilterVariant=ForwardEulerFilter  NVariant=InternalParameters  NCopyVariant=Disabled  FilterICVariant=InternalICsFilter  IntegratorICVariant=InternalICs  ExternalResetVariant=ExternalReset  TRSumVariant=Passthrough  SumFdbkVariant=Disabled  SumVariant=Sum_PID  TsampFilterVariant=InternalTs  TsampNgainVariant=Passthrough  TsampIntegralVariant=Passthrough  ExternalSaturationOutDataTypeStr=Inherit: Same as second input
  Saturation1 : Saturate  UpperLimit=0  LowerLimit=-1  ZeroCross=off
  Saturation2 : Saturate  UpperLimit=5e6  LowerLimit=0  ZeroCross=off
  Saturation4 : Saturate  UpperLimit=1  LowerLimit=0  ZeroCross=off
  Selector : Selector  InputPortWidth=3  IndexOptions=Index vector (dialog)  Indices=[3]  OutputSizes=1
  Selector1 : Selector  InputPortWidth=3  IndexOptions=Index vector (dialog)  Indices=[2]  OutputSizes=1
  Selector2 : Selector  InputPortWidth=4  IndexOptions=Index vector (dialog)  Indices=[3 4]  OutputSizes=1
  Signal Specification : SignalSpecification  Unit=gn
  Signal Specification1 : SignalSpecification  Unit=m/s
  Subtract : Sum
  Subtract1 : Sum  Inputs=+-
  Sum of Elements : Sum  Inputs=+
  Switch1 : Switch  Criteria=u2 > Threshold  Threshold=.1
  Terminator : Terminator
  Unary Minus : UnaryMinus
  Unit Conversion : UnitConversion
  Vector Concatenate2 : Concatenate  NumInputs=4
  axle distance : Constant  Value=VEH.FrontAxlePositionfromCG+VEH.RearAxlePositionfromCG
  div0protect - poly : autolibutils/div0protect - poly  thresh=1  aMode=2
      settings: SourceProductBaseCode=PW,MT,UV,VE,VP
  steer ratio : Gain  Gain=1/18
  wheel radius : Gain  Gain=.3065/4
  zero : Constant  Value=0
  DiffPrsCmd : Outport  VectorParamsAs1DForOutWhenUnconnected=off
  TrqCmd : Outport  Port=2  VectorParamsAs1DForOutWhenUnconnected=off
  wires:
  Vector Concatenate2/1 -> Gain/1  "Reference P"
  Ground/1 -> Vector Concatenate2/2, Vector Concatenate2/1
  Saturation1/1 -> Unary Minus/1
  Gain/1 -> Saturation2/1
  Saturation2/1 -> DiffPrsCmd/1  "DiffPrsCmd"
  Divide3/1 -> Add1/1
  Selector/1 -> Divide3/2
  Logical Operator/1 -> PID Controller/2, Switch1/2
  Switch1/1 -> PID Controller/1
  zero/1 -> Switch1/3
  PID Controller/1 -> Subtract/2
  Add1/1 -> Switch1/1
  axle distance/1 -> Divide3/1
  pqr/1 -> Selector/1
  Compare To Constant2/1 -> Logical Operator/1
  Compare To Constant/1 -> Logical Operator/2
  Abs2/1 -> Compare To Constant2/1
  Steer/1 -> Abs2/1, steer ratio/1
  [xdot] -> Compare To Constant/1
  axayaz/1 -> Selector1/1
  Sum of Elements/1 -> wheel radius/1
  wheel radius/1 -> Signal Specification1/1
  Omega/1 -> Selector2/1, Sum of Elements/1
  Signal Specification1/1 -> [xdot]
  BrkCmd/1 -> Compare To Constant1/1
  GearFdbk/1 -> Compare To Constant3/1
  Compare To Constant3/1 -> Logical Operator/3
  Subtract/1 -> Saturation1/1, Saturation4/1
  Accel/1 -> Compare To Constant4/1
  Compare To Constant4/1 -> Logical Operator/4
  steer ratio/1 -> Add1/2
  Saturation4/1 -> Vector Concatenate2/3
  Selector1/1 -> Unit Conversion/1
  Signal Specification/1 -> Abs3/1
  Abs3/1 -> Dead Zone/1
  Dead Zone/1 -> Subtract/1
  Constant/1 -> TrqCmd/1
  Selector2/1 -> Demux/1
  Demux/1 -> Subtract1/1
  Demux/2 -> Subtract1/2
  Unary Minus/1 -> Vector Concatenate2/4
  Subtract1/1 -> Terminator/1  "wheel speed diff"
  Compare To Constant1/1 -> Logical Operator/5
  Unit Conversion/1 -> Signal Specification/1
  [xdot] -> div0protect - poly/1
  div0protect - poly/1 -> Divide3/3

== system Overtaking_Integrated/Vehicle Plant/Controllers/Brake Controller/Brake Pressure Control ==
  note: 1) Add Subsystem or Model blocks as valid variant choices.
      | 2) You cannot connect blocks at this level. At simulation, connectivity is automatically
      | determined, based on the active variant and port name matching.
  Pref : Inport
  Omega : Inport  Port=2
  <Kappa> : Inport  Port=3
  Bang Bang ABS : Subsystem  VariantControl=1
  Open Loop : Subsystem  VariantControl=0
  BrkPrsCmd : Outport  VectorParamsAs1DForOutWhenUnconnected=off

== system Overtaking_Integrated/Vehicle Plant/Controllers/ECU/Torque Cmd ==
  DiffTrqCmd : Inport
  <Accel> : Inport  Port=2
  EngSpd : Inport  Port=3
  Acc to Torque Request : Gain  Gain=150
  Max : MinMax  Function=max  Inputs=2
  Rev Limiter Control : Subsystem
  Signal Specification : SignalSpecification  Unit=rpm
  Unit Conversion : UnitConversion
  EngTrqCmd : Outport
  wires:
  Signal Specification/1 -> Rev Limiter Control/2(EngSpd)  "EngSpd"
  Unit Conversion/1 -> Signal Specification/1
  EngSpd/1 -> Unit Conversion/1
  <Accel>/1 -> Acc to Torque Request/1
  Acc to Torque Request/1 -> Rev Limiter Control/1(TrqCmd)
  DiffTrqCmd/1 -> Max/1
  Rev Limiter Control/1(TrqCmdRevLimited) -> Max/2
  Max/1 -> EngTrqCmd/1

== system Overtaking_Integrated/Vehicle Plant/Controllers/Transmission Controller/Driver - No Clutch ==
  GearReq : Inport
  Gear : Outport  VectorParamsAs1DForOutWhenUnconnected=off
  wires:
  GearReq/1 -> Gear/1

== system Overtaking_Integrated/Vehicle Plant/Controllers/Transmission Controller/PRNDL Controller ==
  Accel : Inport
  BrkCmd : Inport  Port=2
  Omega : Inport  Port=3  Unit=rad/s
  EngSpd : Inport  Port=4  Unit=rad/s
  GearReq : Inport  Port=5
  Gain : Gain  Gain=.3065/4
  Rate Transition1 : RateTransition  Deterministic=off
  Shift Controller : Stateflow chart  InitFcn=[~] = vehdynicon('vedhynmaneuver',gcb,0)  TreatAsAtomicUnit=on  mask(Shift Scheduler){GearInit=0, pdlVec=[.1 .4 .75 1], upShftTbl=[-1 20 35 40 50 60 70 85; -1 25 45 55 60 65 75 85; -1 30 40 55 65 80 120 150; -1 45 55 65 75 90 150 185], dwnShftTbl=[5 10 15 25 30 40 55 75;4 10 18 25 35 50 65 80;8 12 18 21 55 65 75 85; 10 15 20 25 555 70 80 95], tClutch=.5, tRev=.2, tPark=120, UpGearVec=[ 1  2  3  4  5  6  7 8], DownGearVec=[0 1 2  3  4  5  6  7 ]}
      mask prompts: GearInit "autoblks_shared:autoblkLongitudinalDriver:blkPrm_GearInit"; pdlVec "autoblks_shared:autoblkLongitudinalDriver:blkPrm_pdlVec"; upShftTbl "autoblks_shared:autoblkLongitudinalDriver:blkPrm_upShftTbl"; dwnShftTbl "autoblks_shared:autoblkLongitudinalDriver:blkPrm_dwnShftTbl"; tClutch "autoblks_shared:autoblkLongitudinalDriver:blkPrm_tClutch"; tRev "autoblks_shared:autoblkLongitudinalDriver:blkPrm_tRev"; tPark "autoblks_shared:autoblkLongitudinalDriver:blkPrm_tPark"; UpGearVec "autoblks_shared:autoblkLongitudinalDriver:blkPrm_UpGearVec"; DownGearVec "autoblks_shared:autoblkLongitudinalDriver:blkPrm_DownGearVec"
      mask help: An elementary shift manager which includes a notion of Neutral, Park and Reverse gear logic.
  Signal Specification : SignalSpecification  Unit=rpm
  Signal Specification1 : SignalSpecification  Unit=m/s
  Signal Specification2 : SignalSpecification  Unit=km/hr
  Sum of Elements : Sum  Inputs=+
  Terminator : Terminator
  Unit Conversion : UnitConversion
  Unit Conversion1 : UnitConversion
  Gear : Outport  VectorParamsAs1DForOutWhenUnconnected=off
  wires:
  BrkCmd/1 -> Shift Controller/3(Brake)
  Shift Controller/1(Gear) -> Gear/1
  Gain/1 -> Signal Specification1/1
  Omega/1 -> Sum of Elements/1
  Sum of Elements/1 -> Gain/1
  Shift Controller/2(clutchControl) -> Terminator/1
  Accel/1 -> Shift Controller/2(Accel)
  Signal Specification/1 -> Rate Transition1/1
  EngSpd/1 -> Unit Conversion/1
  Unit Conversion/1 -> Signal Specification/1
  Rate Transition1/1 -> Shift Controller/4(EngSpd)  "EngSpd"
  GearReq/1 -> Shift Controller/1(PRNDL)  "PRNDL"
  Signal Specification1/1 -> Unit Conversion1/1
  Unit Conversion1/1 -> Signal Specification2/1
  Signal Specification2/1 -> Shift Controller/5(VehVel)

== system Overtaking_Integrated/Vehicle Plant/Controllers/Transmission Controller/Paddles ==
  Accel : Inport
  EngSpd : Inport  Port=2  Unit=rad/s
  Add1 : Sum  Inputs=+-+
  Current Gear : UnitDelay  SampleTime=-1  HasFrameUpgradeWarning=on
  Data Type Conversion2 : DataTypeConversion  OutDataTypeStr=double
  Debounce : autolibutils/Debounce  DbcOn_Cnts=10  DbcOff_Cnts=10  aMode=aMode
      settings: SourceProductBaseCode=PW,MT,UV,VE,VP
  Debounce1 : autolibutils/Debounce  DbcOn_Cnts=10  DbcOff_Cnts=10  aMode=aMode
      settings: SourceProductBaseCode=PW,MT,UV,VE,VP
  Demux : Demux  Outputs=2
  Detect Increase2 : simulink/Logic and Bit Operations/Detect Increase  vinit=0.0  OutDataTypeStr=boolean
  Logical Operator1 : Logic  Operator=XOR  Inputs=1  AllPortsSameDT=off  OutDataTypeStr=boolean
  Mux : Mux  Inputs=2
  Switch2 : Switch  Criteria=u2 > Threshold
  Gear : Outport  VectorParamsAs1DForOutWhenUnconnected=off
  wires:
  Debounce/1 -> Mux/1
  Mux/1 -> Detect Increase2/1
  Logical Operator1/1 -> Switch2/2
  Data Type Conversion2/1 -> Demux/1
  Demux/1 -> Add1/1
  Demux/2 -> Add1/2
  Current Gear/1 -> Add1/3, Switch2/3
  Switch2/1 -> Gear/1, Current Gear/1
  Debounce1/1 -> Mux/2
  Add1/1 -> Switch2/1
  Detect Increase2/1 -> Data Type Conversion2/1, Logical Operator1/1
  EngSpd/1 -> Debounce1/1
  Accel/1 -> Debounce/1

== system Overtaking_Integrated/Vehicle Plant/Controllers/Transmission Controller/Transmission Controller ==
  Accel : Inport
  EngSpd : Inport  Port=2  Unit=rad/s
  Omega : Inport  Port=3  Unit=rad/s
  10ms Function-Call Generator : simulink/Ports & Subsystems/Function-Call Generator  sample_time=0.01  numberOfIterations=1  DisallowWideOutput=off
  Data Type Conversion : DataTypeConversion
  First Order Hold : FirstOrderHold  ErrorTolerance=.1
  Rate Transition : RateTransition  Deterministic=off
  Rate Transition1 : RateTransition  Deterministic=off
  Rate Transition2 : RateTransition  Deterministic=off
  Signal Specification : SignalSpecification  Unit=rpm
  TCM : Subsystem
  Unit Conversion : UnitConversion
  Gear : Outport  VectorParamsAs1DForOutWhenUnconnected=off
  wires:
  TCM/1(GearCmd) -> Data Type Conversion/1
  Rate Transition/1 -> TCM/1(AccCmd)
  10ms Function-Call Generator/1 -> TCM/Trigger
  Accel/1 -> Rate Transition/1
  Omega/1 -> Rate Transition2/1
  Rate Transition1/1 -> TCM/2(EngSpd)
  First Order Hold/1 -> Gear/1
  Unit Conversion/1 -> Signal Specification/1
  Signal Specification/1 -> Rate Transition1/1  "EngSpd"
  EngSpd/1 -> Unit Conversion/1
  Data Type Conversion/1 -> First Order Hold/1
  Rate Transition2/1 -> TCM/3(Omega)

== system Overtaking_Integrated/Vehicle Plant/Environment/Ground Feedback/3D Engine ==
  Friction : Inport
  Bus Creator : BusCreator  Inputs=4
  Bus Creator2 : BusCreator  Inputs=4
  Bus Creator3 : BusCreator  Inputs=2
  Bus Selector : BusSelector  OutputSignals=HitLoc
  Data Type Conversion : DataTypeConversion
  Demux : Demux
  Demux1 : Demux
  First Order Hold : FirstOrderHold  ErrorTolerance=1
  Passenger Vehicle Ray Trace Set : sim3dlib/Vehicle Terrain Sensor  Priority=1  ActorTag=EgoVehicle  VehExtEn=Constant  TireRadiiExt=Constant  VehCntrLngthVal=0  TireRadiiVal=0  VehRayLngth=10  LfRayLngth=20  RfRayLngth=20  LrRayLngth=20  RrRayLngth=20  VehRayOffset=0  LfRayOffset=-1  RfRayOffset=-1  LrRayOffset=-1  RrRayOffset=-1  VehEn=on  LfEn=on  RfEn=on  LrEn=on  RrEn=on  DbgEn=off  Ts=dt  aMode=2
      settings: SourceProductBaseCode=DR,UV,VE
  Range Limiter : Saturate  UpperLimit=1e3  LowerLimit=-1e3  ZeroCross=off
  Reshape10 : Reshape  OutputDimensionality=Row vector (2-D)
  Selector1 : Selector  InputPortWidth=5  IndexOptions=Index vector (dialog)  Indices=[2:5]  OutputSizes=1
  Signal Specification : SignalSpecification  Unit=m
  Signal Specification1 : SignalSpecification  Unit=1
  Terminator1 : Terminator
  Terminator2 : Terminator
  Zend Select : Selector  NumberOfDimensions=2  InputPortWidth=3  IndexOptions=Select all,Index vector (dialog)  Indices=[1 3],3  OutputSizes=1,1
  Ground : Outport  VectorParamsAs1DForOutWhenUnconnected=off
  wires:
  Zend Select/1 -> Reshape10/1
  Bus Selector/1 -> Range Limiter/1  "<HitLoc>"
  Passenger Vehicle Ray Trace Set/2 -> Terminator1/1
  Passenger Vehicle Ray Trace Set/3 -> Terminator2/1
  Reshape10/1 -> Selector1/1
  Passenger Vehicle Ray Trace Set/1 -> Bus Selector/1
  Selector1/1 -> Data Type Conversion/1
  Demux/2 -> Bus Creator/2  "G_FR_z"
  Demux/1 -> Bus Creator/1  "G_FL_z"
  Demux/4 -> Bus Creator/4  "G_RR_z"
  Demux/3 -> Bus Creator/3  "G_RL_z"
  Signal Specification/1 -> Demux/1
  Signal Specification1/1 -> Demux1/1
  Demux1/1 -> Bus Creator2/1  "mu_FL"
  Bus Creator/1 -> Bus Creator3/1  "z"
  Demux1/3 -> Bus Creator2/3  "mu_RL"
  Demux1/4 -> Bus Creator2/4  "mu_RR"
  Demux1/2 -> Bus Creator2/2  "mu_FR"
  Bus Creator2/1 -> Bus Creator3/2  "mu"
  Bus Creator3/1 -> Ground/1
  Range Limiter/1 -> Zend Select/1
  First Order Hold/1 -> Signal Specification/1
  Data Type Conversion/1 -> First Order Hold/1
  Friction/1 -> Signal Specification1/1

== system Overtaking_Integrated/Vehicle Plant/Environment/Ground Feedback/Constant ==
  Friction : Inport
  Bus Creator : BusCreator  Inputs=4
  Bus Creator2 : BusCreator  Inputs=4
  Bus Creator3 : BusCreator  Inputs=2
  Constant1 : Constant  Value=zeros(4,1)
  Demux : Demux
  Demux1 : Demux
  Signal Specification : SignalSpecification  Unit=m
  Signal Specification1 : SignalSpecification  Unit=1
  Ground : Outport  VectorParamsAs1DForOutWhenUnconnected=off
  wires:
  Constant1/1 -> Signal Specification/1
  Signal Specification/1 -> Demux/1
  Demux/4 -> Bus Creator/4  "G_RR_z"
  Demux/1 -> Bus Creator/1  "G_FL_z"
  Demux/3 -> Bus Creator/3  "G_RL_z"
  Demux/2 -> Bus Creator/2  "G_FR_z"
  Bus Creator/1 -> Bus Creator3/1  "z"
  Demux1/3 -> Bus Creator2/3  "mu_RL"
  Demux1/4 -> Bus Creator2/4  "mu_RR"
  Demux1/1 -> Bus Creator2/1  "mu_FL"
  Demux1/2 -> Bus Creator2/2  "mu_FR"
  Bus Creator2/1 -> Bus Creator3/2  "mu"
  Friction/1 -> Signal Specification1/1
  Signal Specification1/1 -> Demux1/1
  Bus Creator3/1 -> Ground/1
